simulink model "PID_reference_model"  (R2020b)
settings: Solver=VariableStepAuto  StartTime=0.0  StopTime=10.0  RelTol=1e-3
values from neighbouring files (symbols this model uses):
  Kd = 10.0    [PID_data_dict.sldd]    (also in W2ques3_code.m = 10)
  Ki = 50.0    [PID_data_dict.sldd]    (also in W2ques3_code.m = 50)
  Kp = 100.0    [PID_data_dict.sldd]    (also in W2ques3_code.m = 100)
settings Model: Creator=sneha  LastModifiedBy=sneha
settings DataIOCC: SaveOutput=off  SaveTime=off

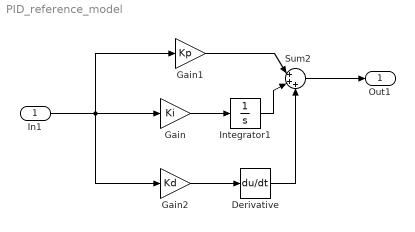
== system PID_reference_model ==
  In1 : Inport  OutDataTypeStr=double  PortDimensions=1  SampleTime=0
  Derivative : Derivative
  Gain : Gain  Gain=Ki
  Gain1 : Gain  Gain=Kp
  Gain2 : Gain  Gain=Kd
  Integrator1 : Integrator
  Sum2 : Sum  Inputs=|+++
  Out1 : Outport  OutDataTypeStr=double  PortDimensions=1  SampleTime=0
  wires:
  Gain/1 -> Integrator1/1
  Gain1/1 -> Sum2/1
  Integrator1/1 -> Sum2/2
  In1/1 -> Gain2/1, Gain1/1, Gain/1
  Sum2/1 -> Out1/1
  Gain2/1 -> Derivative/1
  Derivative/1 -> Sum2/3
